simulink model "rayleighAWGN"  (Simulink 7.4)
settings: Solver=FixedStepDiscrete  StartTime=0  StopTime=8.1  RelTol=1e-3
PreLoadFcn:
  | set(0,'ShowHiddenHandles','on');
  | if strcmp(get(findobj('Tag','Powerslider'),'Enable'),'on')
  |    simulink('open');
  |    set(0,'ShowHiddenHandles','on')
  |    h=findobj('Tag','MainFigureOfVlabs2');
  |    set(h,'Visible','off');
  | end
InitFcn:
  | set(0,'ShowHiddenHandles','on')
  | if strcmp(get(findobj('Tag','Powerslider'),'Enable'),'off')
  | 
  | seed_binary = 12345;
  | M=4;
  | EbNo=5;
  | randseed_AWGN = 12351;
  | seed_rayleigh = 12349;
  | maxNumErrs=inf;
  | maxNumBits=inf;
  | Ps=1;
  | SymbolPeriod=1e-6;
  | probOfZero=0.5;
  | 
  | end
StopFcn:
  | % set_param('vrWorldVlab2','simulationcommand','continue');
  | try
  | 
  | 
  | setcarpos( 90 );
  | 
  | HH=findobj(findobj('Tag','MainFigureOfVlabs2'),'Type','uicontrol');
  | for i=1:length(HH)
  |   set(HH(i),'enable','on');
  |   if strcmp(get(HH(i),'Tag'),'Pausebtn' )
  |       set(HH(i),'enable','off');
  |   end
  |   if strcmp(get(HH(i),'Tag'),'Stopbtn' )
  |       set(HH(i),'enable','off');
  |   end
  | end
  | 
  | 
  | 
  | 
  |   set(findobj('Tag','ShowViewerBtnMenu'),'Enable','on');
  |   set(findobj('Tag','DemoPlayMenuBtn'),'Enable','on');
  | 
  | showGains=get(findobj('Tag','Fdcheck'),'Value'); %show gains..
  | if showGains
  | global globalTgain;
  | global globalPgain;
  | global globalRgain;
  | global ShadowvaryDB;
  | 
  | figure;
  | subplot(3,2,1);
  | plot(0:180/199:180,10*log10(globalTgain));
  | xlabel('distance - (m)');
  | ylabel('dB');
  | title('Transmitter Antenna Gain');
  | 
  | subplot(3,2,2);
  | plot(0:180/199:180,-10*log10(globalPgain));
  | xlabel('distance - (m)');
  | ylabel('dB');
  | title('Path Loss');
  | 
  | subplot(3,2,3);
  | plot(0:180/199:180,10*log10(globalRgain));
  | xlabel('distance - (m)');
  | ylabel('dB');
  | title('Receiver Antenna Gain');
  | 
  | subplot(3,2,4);
  | plot(0:180/199:180,ShadowvaryDB);
  | xlabel('distance - (m)');
  | ylabel('dB');
  | title('Shadowing Losses');
  | 
  | subplot(3,2,5:6);
  | plot(0:180/199:180,-10*log10(globalPgain)+10*log10(globalRgain)+10*log10(globalTgain)+ShadowvaryDB);
  | xlabel('distance - (m)');
  | ylabel('dB');
  | title('Aggregate Gains');
  | 
  | end
  | 
  | showTIR=get(findobj('Tag','TIRcheck'),'Value'); %show TIR..
  | showPDP=get(findobj('Tag','PDPcheck'),'Value'); %show PDP..
  | 
  | 
  | if showTIR
  | n=length(ImResp);
  | x3=0:180/(n-1):180;
  | y3=10*log10(ImResp);
  | else
  | x3=1;
  | y3=1;
  | end
  | 
  | if showPDP
  | global Delays;
  | global Gains;
  | x2=Delays;
  | y2=Gains;
  | else
  | x2=1;
  | y2=1;
  | end
  | 
  | 
  | x1=1;
  | y1=1;
  | 
  | global globalT;
  | 
  | report([1 0 showPDP showTIR], ...
  |            {'minimum BER' 'minimum SER' 'Average Fade Duration' 'Level Crossing Frequency'}, ...
  |            {BER(1) SER(1) 3 4}, ...
  |            {x1 abs(y1)},...
  |            {x2 y2},...
  |            {x3 y3 globalT}  );
  | 
  | catch MException
  | end
undefined symbols (not defined in the file or in its folder): j
libraries: commchan3 x2, commdigbbndpm3 x2, commutil2 x2, commsink2 x2, dspstat3 x1, commrandsrc2 x1
CloseFcn:
  | set(0,'ShowHiddenHandles','on')
  | if strcmp(get(findobj('Tag','Powerslider'),'Enable'),'on')
  | simulink('close');
  | 
  | orient landscape;
  | delete('blocks.png');
  | print -srayleighAWGN -dpng 'blocks.png'
  | 
  | RGB = imread('blocks.png');
  | RGB = imrotate(RGB,-90);
  | RGB = imresize(RGB, [241 348]);
  | imwrite(RGB,'blocks.png');
  | 
  | set(0,'ShowHiddenHandles','on')
  | 
  | h1=findobj('Tag','MainFigureOfVlabs2');
  | set(h1,'Visible','on');
  | 
  | h=findobj(h1,'Type','axes');
  |        image(RGB,'Parent',h);
  |        set(h,'XTick',[]);
  |        set(h,'YTick',[]);
  | end
settings Model: Creator=cls  LastModifiedBy=Administrator
settings OptimizationCC: InlineInvariantSignals=on  InitFltsAndDblsToZero=on  EfficientMapNaN2IntZero=off
settings DebuggingCC: SaveWithParameterizedLinksMsg=none  SignalResolutionControl=TryResolveAllWithWarning  MultiTaskDSMMsg=warning  MultiTaskCondExecSysMsg=none  StrictBusMsg=None
settings RTWCC: IncludeERTFirstTime=on
settings GRTTargetCC: TargetFcnLib=ansi_tfl_tmw.mat

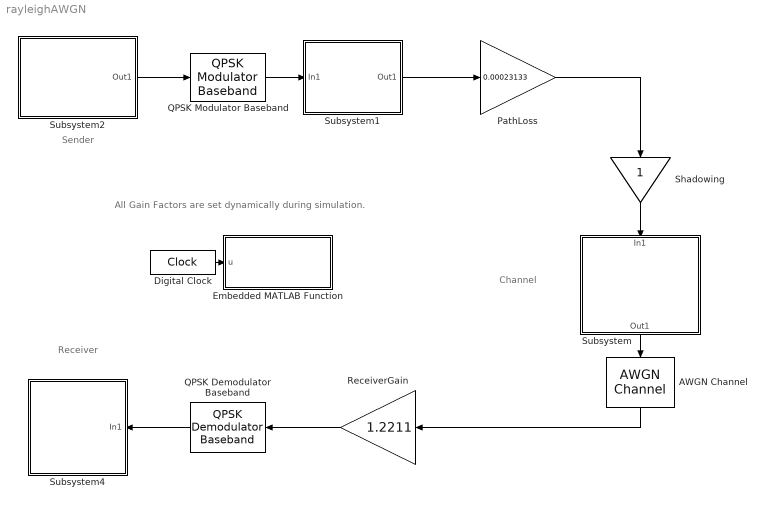
== system rayleighAWGN ==
  note: Sender
  note: Receiver
  note: Channel
  note: All Gain Factors are set
      | dynamically during simulation.
  AWGN Channel : commchan3/AWGN Channel  SystemSampleTime=-1  seed=randseed_AWGN  noiseMode="Signal to noise ratio  (SNR)"  EbNodB=EbNo  EsNodB=10  SNRdB=0  bitsPerSym=log2(M)  Ps=Ps  Tsym=SymbolPeriod  variance=1
  Digital Clock : DigitalClock  SampleTime=0.1
  Embedded MATLAB Function : Stateflow chart
  PathLoss : Gain  Gain=0.00023133  ParameterDataType=fixdt(1, 16)  ParameterScaling=2^0  OutDataType=fixdt(1, 16)  OutScaling=2^0
  QPSK Demodulator Baseband : commdigbbndpm3/QPSK Demodulator Baseband  DialogController=commDDGCreate  DialogControllerArgs=DataTag0  Ph=pi/4  Dec=Gray  OutType=Bit  DecType=Hard decision  VarSource=Dialog  Variance=1  outDtype1=double  outDtype2=double  derotateFactorWordLen=16
  QPSK Modulator Baseband : commdigbbndpm3/QPSK Modulator Baseband  DialogController=commDDGCreate  DialogControllerArgs=DataTag1  SystemSampleTime=-1  InType=Bit  Enc=Gray  Ph=pi/4  outDtype=double  outWordLen=16  outUDDataType=sfix(16)  outFracLenMode=Best precision  outFracLen=15
  ReceiverGain : Gain  Gain=1.2211  ParameterDataType=fixdt(1, 16)  ParameterScaling=2^0  OutDataType=fixdt(1, 16)  OutScaling=2^0
  Shadowing : Gain  ParameterDataType=fixdt(1, 16)  ParameterScaling=2^0  OutDataType=fixdt(1, 16)  OutScaling=2^0
  Subsystem : Subsystem
      mask Display: fprintf('Fading\nprocedure')
  Subsystem1 : Subsystem
      mask Display: fprintf('Sender\nGain')
  Subsystem2 : Subsystem
      mask Display: fprintf('Signal\nSource')
  Subsystem4 : Subsystem
      mask Display: fprintf('Received\nSignal')
  wires:
  QPSK Modulator Baseband/1 -> Subsystem1/1(In1)
  QPSK Demodulator Baseband/1 -> Subsystem4/1(In1)
  ReceiverGain/1 -> QPSK Demodulator Baseband/1
  Subsystem2/1(Out1) -> QPSK Modulator Baseband/1
  Shadowing/1 -> Subsystem/1(In1)
  Subsystem/1(Out1) -> AWGN Channel/1
  Subsystem1/1(Out1) -> PathLoss/1
  AWGN Channel/1 -> ReceiverGain/1
  Digital Clock/1 -> Embedded MATLAB Function/1(u)
  PathLoss/1 -> Shadowing/1

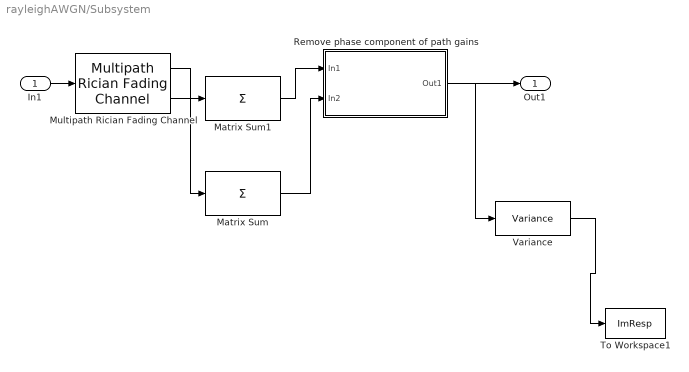
== system rayleighAWGN/Subsystem ==
  In1 : Inport
  Matrix Sum : Sum  Inputs=+  CollapseMode=Specified dimension  CollapseDim=2  OutDataType=sfix(16)  OutScaling=2^-10
  Matrix Sum1 : Sum  Inputs=+  CollapseMode=Specified dimension  CollapseDim=2  OutDataType=sfix(16)  OutScaling=2^-10
  Multipath Rician Fading Channel : commchan3/Multipath Rician Fading Channel  SystemSampleTime=-1  K=26  fdLOS=-65.481  thetaLOS=0  maxDopplerShift=74.0728  spectrumType=Jakes  sigmaGaussian=1/sqrt(2)  coeffRounded=[1 -1.72 0.785]  freqMinMaxRJakes=[0 1]  freqMinMaxAJakes=[0 1]  sigmaGaussian1=1/sqrt(2)  sigmaGaussian2=1/sqrt(2)  centerFreqGaussian1=0  centerFreqGaussian2=0  gainGaussian1=0.5  gainGaussian2=0.5  coeffBell=9  dopplerSpectrum=doppler.jakes  pathDelays=[0]  avgPathGaindB=[0]  normalizePathGains=on  seed=73  enableProbe=0  openVisAtStart=off  outPathGains=on  outDelay=off
  Remove phase component of path gains : Subsystem
      mask Display: disp('Remove phase component\nof path gains')
  To Workspace1 : ToWorkspace  VariableName=ImResp  SampleTime=-1  SaveFormat=Array
  Variance : dspstat3/Variance  DialogController=dspDDGCreate  DialogControllerArgs=DataTag2  run=off  reset_popup=None  directionMode=Each column  dimension=1  treatSBRowAsCol=on  roiEnable=off  roiType=Rectangles  roiPortion=Entire ROI  roiOutput=Individual statistics for each ROI  roiFlag=off  roundingMode=Floor  overflowMode=off
  Out1 : Outport
  wires:
  In1/1 -> Multipath Rician Fading Channel/1
  Remove phase component of path gains/1(Out1) -> Out1/1, Variance/1
  Variance/1 -> To Workspace1/1
  Multipath Rician Fading Channel/1 -> Matrix Sum/1
  Matrix Sum/1 -> Remove phase component of path gains/2(In2)
  Multipath Rician Fading Channel/2 -> Matrix Sum1/1
  Matrix Sum1/1 -> Remove phase component of path gains/1(In1)

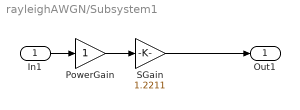
== system rayleighAWGN/Subsystem1 ==
  In1 : Inport
  PowerGain : Gain  ParameterDataType=fixdt(1, 16)  ParameterScaling=2^0  OutDataType=fixdt(1, 16)  OutScaling=2^0
  SGain : Gain  Gain=1.2211  ParameterDataType=fixdt(1, 16)  ParameterScaling=2^0  OutDataType=fixdt(1, 16)  OutScaling=2^0
  Out1 : Outport
  wires:
  PowerGain/1 -> SGain/1
  SGain/1 -> Out1/1
  In1/1 -> PowerGain/1

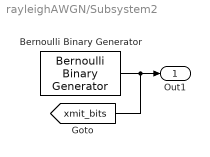
== system rayleighAWGN/Subsystem2 ==
  Bernoulli Binary Generator : commrandsrc2/Bernoulli Binary Generator  DialogController=commDDGCreate  DialogControllerArgs=DataTag3  SystemSampleTime=-1  P=probOfZero  seed=seed_binary  Ts=SymbolPeriod/log2(M)  frameBased=on  sampPerFrame=100*log2(M)  orient=off  outDataType=double
  Out1 : Outport
  tag scope: xmit_bits=global
  wires:
  Bernoulli Binary Generator/1 -> [xmit_bits], Out1/1

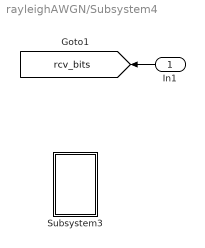
== system rayleighAWGN/Subsystem4 ==
  In1 : Inport
  Subsystem3 : Subsystem
  tag scope: rcv_bits=global
  wires:
  In1/1 -> [rcv_bits]

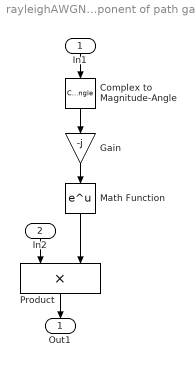
== system rayleighAWGN/Subsystem/Remove phase component of path gains ==
  In1 : Inport  OutDataType=sfix(16)  OutScaling=2^0
  In2 : Inport  Port=2  OutDataType=sfix(16)  OutScaling=2^0
  Complex to Magnitude-Angle : ComplexToMagnitudeAngle  Output=Angle
  Gain : Gain  Gain=-j  ParameterDataType=sfix(16)  ParameterScaling=2^0  OutDataType=sfix(16)  OutScaling=2^0
  Math Function : Math  OutDataType=sfix(16)  OutScaling=2^0  SaturateOnIntegerOverflow=on
  Product : Product  OutDataType=sfix(16)  OutScaling=2^0  RndMeth=Zero
  Out1 : Outport  OutDataType=sfix(16)  OutScaling=2^0
  wires:
  Complex to Magnitude-Angle/1 -> Gain/1
  Gain/1 -> Math Function/1
  Math Function/1 -> Product/2
  In1/1 -> Complex to Magnitude-Angle/1
  In2/1 -> Product/1
  Product/1 -> Out1/1

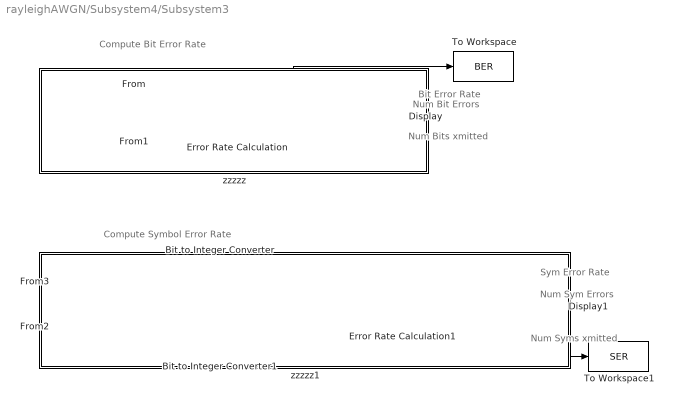
== system rayleighAWGN/Subsystem4/Subsystem3 ==
  note: Num Syms xmitted
  note: Num Sym Errors
  note: Sym Error Rate
  note: Compute Symbol Error Rate
  note: Compute Bit Error Rate
  note: Num Bits xmitted
  note: Num Bit Errors
  note: Bit Error Rate
  Bit to Integer Converter : commutil2/Bit to Integer Converter  nbits=log2(M)  bitOrder=MSB first  signedOutputValues=Unsigned  outDtype=Inherit via internal rule  outDtypeSigned=Inherit via internal rule
  Bit to Integer Converter1 : commutil2/Bit to Integer Converter  nbits=log2(M)  bitOrder=MSB first  signedOutputValues=Unsigned  outDtype=Inherit via internal rule  outDtypeSigned=Inherit via internal rule
  Display : Display
  Display1 : Display
  Error Rate Calculation : commsink2/Error Rate Calculation  N=0  st_delay=0  cp_mode=Entire frame  subframe=[]  PMode=Port  WsName=BER  RsMode2=off  stop=off  numErr=maxNumErrs  maxBits=maxNumBits
  Error Rate Calculation1 : commsink2/Error Rate Calculation  N=0  st_delay=0  cp_mode=Entire frame  subframe=[]  PMode=Port  WsName=ErrorVec  RsMode2=off  stop=on  numErr=maxNumErrs  maxBits=maxNumBits
  To Workspace : ToWorkspace  VariableName=BER  SampleTime=-1  SaveFormat=Array
      settings: MaxDataPoints=1
  To Workspace1 : ToWorkspace  VariableName=SER  SampleTime=-1  SaveFormat=Array
      settings: MaxDataPoints=1
  zzzzz : Subsystem
      mask Display: disp('')
  zzzzz1 : Subsystem
      mask Display: disp('')
  wires:
  Bit to Integer Converter1/1 -> Error Rate Calculation1/2
  Bit to Integer Converter/1 -> Error Rate Calculation1/1
  Error Rate Calculation1/1 -> To Workspace1/1, Display1/1
  [xmit_bits] -> Bit to Integer Converter/1
  [rcv_bits] -> Bit to Integer Converter1/1
  [rcv_bits] -> Error Rate Calculation/2
  [xmit_bits] -> Error Rate Calculation/1
  Error Rate Calculation/1 -> Display/1, To Workspace/1

== system rayleighAWGN/Subsystem4/Subsystem3/zzzzz ==

== system rayleighAWGN/Subsystem4/Subsystem3/zzzzz1 ==

== matlab function Embedded MATLAB Function ==
  data: u input double
function ChangeParam(u) %#eml

eml.extrinsic('set_param');
eml.extrinsic('num2str');
eml.extrinsic('timevary');
eml.extrinsic('vrworld');
eml.extrinsic('vrnode');
eml.extrinsic('getfield');
eml.extrinsic('setfield');
eml.extrinsic('setcarpos');


[Tgain Sgain Pgain Rgain SNRdB K Fd avPathG pathDelays carpos]=timevary(u);

set_param('rayleighAWGN/Subsystem1/SGain','Gain',num2str(sqrt(Tgain)));
set_param('rayleighAWGN/Shadowing','Gain',num2str(sqrt(Sgain)));
set_param('rayleighAWGN/PathLoss','Gain',num2str(sqrt(Pgain)));

set_param('rayleighAWGN/ReceiverGain','Gain',num2str(sqrt(Rgain)));
set_param('rayleighAWGN/AWGN Channel','SNRdB',num2str(SNRdB));
set_param('rayleighAWGN/Subsystem/Multipath Rician Fading Channel','K',num2str(K));
set_param('rayleighAWGN/Subsystem/Multipath Rician Fading Channel','fdLOS',num2str(Fd));
set_param('rayleighAWGN/Subsystem/Multipath Rician Fading Channel','avgPathGaindB',['[' num2str(avPathG) ']']);
set_param('rayleighAWGN/Subsystem/Multipath Rician Fading Channel','pathDelays',['[' num2str(pathDelays) ']']);

setcarpos(carpos);
